simulink model "Project_ESC_System_Harness"  (R2023a)
settings: Solver=FixedStepDiscrete  StartTime=0.0  StopTime=2  FixedStep=0.02  RelTol=1e-3
settings Model: DataDictionary=Project_ESC_Data_Dictionary.sldd  Creator=User  LastModifiedBy=User
settings DataIOCC: ExternalInput=ds.getElement('ESC_On_Off'),ds.getElement('Velocity_of_Car'),ds.getElement('Radius'),ds.getElement('Steering_Angle_Sensor')  LoadExternalInput=on  TimeSaveName=MIL_tout  OutputSaveName=MIL_yout  ReturnWorkspaceOutputsName=MIL_out
settings OptimizationCC: BlockReduction=off  DefaultParameterBehavior=Inlined  UseDivisionForNetSlopeComputation=on  EnhancedBackFolding=on  PassReuseOutputArgsAs=Individual arguments  EfficientFloat2IntCast=on  LifeSpan=inf  OptimizeBlockOrder=speed  DifferentSizesBufferReuse=on  OptimizationCustomize=off  EfficientTunableParamExpr=on
settings DebuggingCC: SignalInfNanChecking=error  SignalRangeChecking=error  ReadBeforeWriteMsg=EnableAllAsError  WriteAfterWriteMsg=EnableAllAsError  WriteAfterReadMsg=EnableAllAsError  AlgebraicLoopMsg=error  ArtificialAlgebraicLoopMsg=error  SaveWithDisabledLinksMsg=error  SaveWithParameterizedLinksMsg=error  BlockPriorityViolationMsg=error  SolverPrmCheckMsg=error  InheritedTsInSrcMsg=error  SingleTaskRateTransMsg=error  TasksWithSamePriorityMsg=error  SigSpecEnsureSampleTimeMsg=error  CheckMatrixSingularityMsg=error  IntegerOverflowMsg=error  ParameterUnderflowMsg=error  ParameterPrecisionLossMsg=none  ParameterTunabilityLossMsg=error  UnderSpecifiedDataTypeMsg=error  UnnecessaryDatatypeConvMsg=warning  VectorMatrixConversionMsg=error  SignalLabelMismatchMsg=error  UnconnectedInputMsg=error  UnconnectedOutputMsg=error  UnconnectedLineMsg=error  SFcnCompatibilityMsg=error  UniqueDataStoreMsg=error  BusObjectLabelMismatch=error  RootOutportRequireBusObject=error  AssertControl=DisableAll  ModelReferenceIOMsg=error  ModelReferenceIOMismatchMessage=error  UnknownTsInhSupMsg=error  ModelReferenceDataLoggingMessage=error  StateNameClashWarn=warning  StrictBusMsg=ErrorOnBusTreatedAsVector  NonBusSignalsTreatedAsBus=error  SFInvalidInputDataAccessInChartInitDiag=error  SFTransitionOutsideNaturalParentDiag=error  SFUnreachableExecutionPathDiag=error  SFUndirectedBroadcastEventsDiag=error  SFTransitionActionBeforeConditionDiag=error  SFTemporalDelaySmallerThanSampleTimeDiag=error  SFSelfTransitionDiag=error  SFExecutionAtInitializationDiag=error  IntegerSaturationMsg=error  VariantConditionMismatch=error
settings SFSimCC: CompileTimeRecursionLimit=0  EnableRuntimeRecursion=off  MATLABDynamicMemAlloc=off
settings RTWCC: Description=Embedded Coder  SystemTargetFile=ert.tlc  GenCodeOnly=on  TemplateMakefile=ert_default_tmf  GenerateReport=on  IncludeHyperlinkInReport=on  LaunchReport=on  GenerateTraceInfo=on  GenerateTraceReport=on  GenerateTraceReportSl=on  GenerateTraceReportEml=on
settings CodeAppCC: ForceParamTrailComments=on  IgnoreCustomStorageClasses=off  OperatorAnnotations=on  SimulinkDataObjDesc=on  SFDataObjDesc=on  MATLABFcnDesc=on  MangleLength=5  InsertBlockDesc=on  ReqsInCode=on
settings ERTTargetCC: TargetLangStandard=C99 (ISO)  UtilityFuncGeneration=Shared location  GenerateSampleERTMain=on  IncludeMdlTerminateFcn=off  SuppressErrorStatus=on  SupportAbsoluteTime=off  SupportNonFinite=off  ParenthesesLevel=Standards  CastingMode=Standards  GenerateSharedConstants=off  InlinedParameterPlacement=NonHierarchical  ERTCustomFileTemplate=example_file_process.tlc  PreserveExpressionOrder=on  SuppressUnreachableDefaultCases=off  EnableSignedLeftShifts=off  EnableSignedRightShifts=off
settings ConfigComp: CovMetricSettings=dcmwe  DVMode=DesignErrorDetection  DVTestSuiteOptimization=Auto  DVDetectOutOfBounds=on  DVModelReferenceHarness=on  DVHarnessSource=Signal Editor

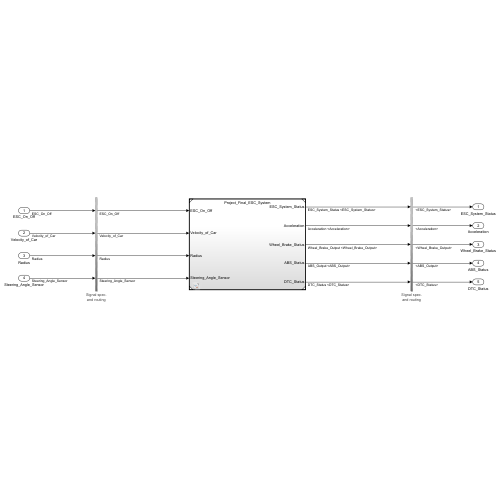
[thumbnail: Simulink's stored preview of the top-level diagram]
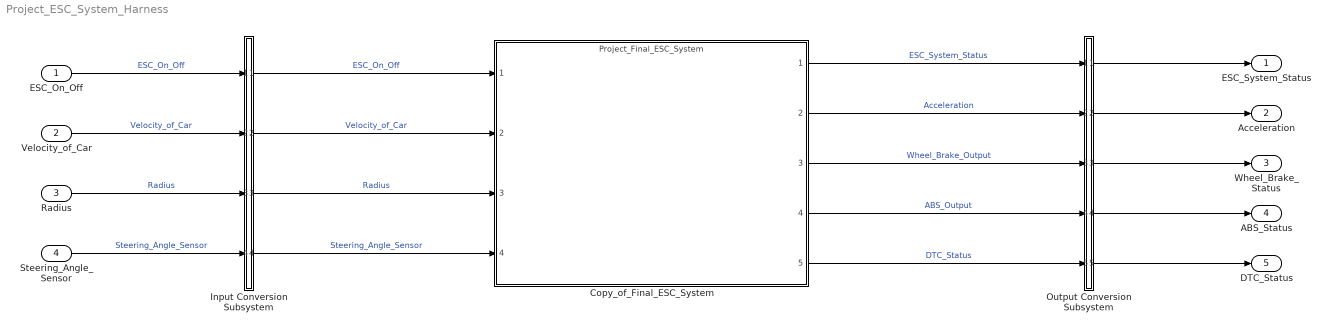
== system Project_ESC_System_Harness ==
  ESC_On_Off : Inport  OutDataTypeStr=boolean  PortDimensions=[1]  SampleTime=0.02
  Velocity_of_Car : Inport  Port=2  OutDataTypeStr=single  PortDimensions=[1]  SampleTime=0.02
  Radius : Inport  Port=3  OutDataTypeStr=single  PortDimensions=[1]  SampleTime=0.02
  Steering_Angle_Sensor : Inport  Port=4  OutDataTypeStr=single  PortDimensions=[1]  SampleTime=0.02
  Copy_of_Final_ESC_System : ModelReference  ModelNameDialog=Project_Final_ESC_System.slx  SimulationMode=Normal  ModelReferenceVersion=1.907
  Input Conversion Subsystem : Subsystem  Tag=__SLT_ICS__  Description=|
      | Signal spec.
      | and routing
      settings: AttributesFormatString=%<Description>
  Output Conversion Subsystem : Subsystem  Tag=__SLT_OCS__  Description=|
      | Signal spec.
      | and routing
      settings: AttributesFormatString=%<Description>
  ESC_System_Status : Outport
  Acceleration : Outport  Port=2
  Wheel_Brake_Status : Outport  Port=3
  ABS_Status : Outport  Port=4
  DTC_Status : Outport  Port=5
  wires:
  ESC_On_Off/1 -> Input Conversion Subsystem/1(Inport_1)  "ESC_On_Off"
  Velocity_of_Car/1 -> Input Conversion Subsystem/2(Inport_2)  "Velocity_of_Car"
  Radius/1 -> Input Conversion Subsystem/3(Inport_3)  "Radius"
  Steering_Angle_Sensor/1 -> Input Conversion Subsystem/4(Inport_4)  "Steering_Angle_Sensor"
  Output Conversion Subsystem/1(Outport_1) -> ESC_System_Status/1
  Output Conversion Subsystem/2(Outport_2) -> Acceleration/1
  Output Conversion Subsystem/3(Outport_3) -> Wheel_Brake_Status/1
  Output Conversion Subsystem/4(Outport_4) -> ABS_Status/1
  Output Conversion Subsystem/5(Outport_5) -> DTC_Status/1
  Input Conversion Subsystem/1(Outport_1) -> Copy_of_Final_ESC_System/1  "ESC_On_Off"
  Input Conversion Subsystem/2(Outport_2) -> Copy_of_Final_ESC_System/2  "Velocity_of_Car"
  Input Conversion Subsystem/3(Outport_3) -> Copy_of_Final_ESC_System/3  "Radius"
  Input Conversion Subsystem/4(Outport_4) -> Copy_of_Final_ESC_System/4  "Steering_Angle_Sensor"
  Copy_of_Final_ESC_System/1 -> Output Conversion Subsystem/1(Inport_1)  "ESC_System_Status"
  Copy_of_Final_ESC_System/2 -> Output Conversion Subsystem/2(Inport_2)  "Acceleration"
  Copy_of_Final_ESC_System/3 -> Output Conversion Subsystem/3(Inport_3)  "Wheel_Brake_Output"
  Copy_of_Final_ESC_System/4 -> Output Conversion Subsystem/4(Inport_4)  "ABS_Output"
  Copy_of_Final_ESC_System/5 -> Output Conversion Subsystem/5(Inport_5)  "DTC_Status"

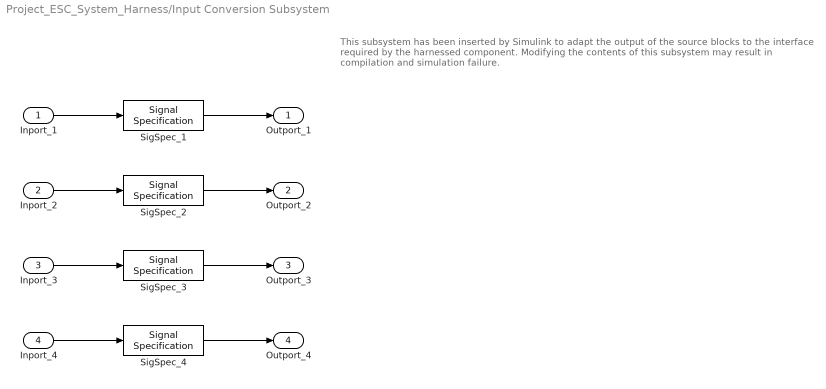
== system Project_ESC_System_Harness/Input Conversion Subsystem ==
  note: This subsystem has been inserted by Simulink to adapt the output of the source blocks to the interface required by the harnessed component.
      |  Modifying the contents of this subsystem may result in compilation and simulation failure.
  Inport_1 : Inport
  Inport_2 : Inport  Port=2
  Inport_3 : Inport  Port=3
  Inport_4 : Inport  Port=4
  SigSpec_1 : SignalSpecification  OutDataTypeStr=boolean  Dimensions=[1]  SampleTime=0.02
  SigSpec_2 : SignalSpecification  OutDataTypeStr=single  Dimensions=[1]  SampleTime=0.02
  SigSpec_3 : SignalSpecification  OutDataTypeStr=single  Dimensions=[1]  SampleTime=0.02
  SigSpec_4 : SignalSpecification  OutDataTypeStr=single  Dimensions=[1]  SampleTime=0.02
  Outport_1 : Outport
  Outport_2 : Outport  Port=2
  Outport_3 : Outport  Port=3
  Outport_4 : Outport  Port=4
  wires:
  SigSpec_1/1 -> Outport_1/1
  Inport_1/1 -> SigSpec_1/1
  SigSpec_2/1 -> Outport_2/1
  Inport_2/1 -> SigSpec_2/1
  SigSpec_3/1 -> Outport_3/1
  Inport_3/1 -> SigSpec_3/1
  SigSpec_4/1 -> Outport_4/1
  Inport_4/1 -> SigSpec_4/1

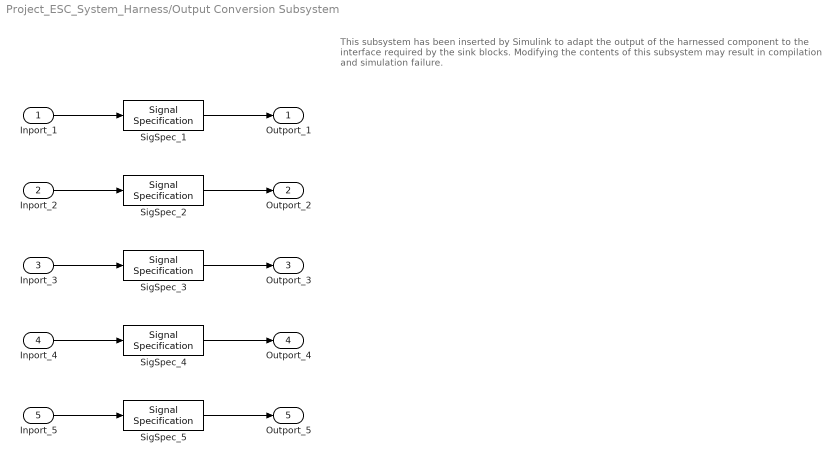
== system Project_ESC_System_Harness/Output Conversion Subsystem ==
  note: This subsystem has been inserted by Simulink to adapt the output of the harnessed component to the interface required by the sink blocks.
      |  Modifying the contents of this subsystem may result in compilation and simulation failure.
  Inport_1 : Inport
  Inport_2 : Inport  Port=2
  Inport_3 : Inport  Port=3
  Inport_4 : Inport  Port=4
  Inport_5 : Inport  Port=5
  SigSpec_1 : SignalSpecification  OutDataTypeStr=boolean  Dimensions=[1]  SampleTime=0.02
  SigSpec_2 : SignalSpecification  OutDataTypeStr=single  Dimensions=[1]  SampleTime=0.02
  SigSpec_3 : SignalSpecification  OutDataTypeStr=single  Dimensions=[1]  SampleTime=0.02
  SigSpec_4 : SignalSpecification  OutDataTypeStr=boolean  Dimensions=[1]  SampleTime=0.02
  SigSpec_5 : SignalSpecification  OutDataTypeStr=single  Dimensions=[1]  SampleTime=0.02
  Outport_1 : Outport
  Outport_2 : Outport  Port=2
  Outport_3 : Outport  Port=3
  Outport_4 : Outport  Port=4
  Outport_5 : Outport  Port=5
  wires:
  Inport_1/1 -> SigSpec_1/1
  SigSpec_1/1 -> Outport_1/1
  Inport_2/1 -> SigSpec_2/1
  SigSpec_2/1 -> Outport_2/1
  Inport_3/1 -> SigSpec_3/1
  SigSpec_3/1 -> Outport_3/1
  Inport_4/1 -> SigSpec_4/1
  SigSpec_4/1 -> Outport_4/1
  Inport_5/1 -> SigSpec_5/1
  SigSpec_5/1 -> Outport_5/1
